simulink model "sgMdl_IO723_CANLoopback"  (R2024b)
settings: Solver=FixedStepAuto  StartTime=0.0  StopTime=inf  RelTol=1e-3
undefined symbols (not defined in the file): sgrestbus
libraries: speedgoatlib_IO723 x3
Description:
  | IO723 - CAN Loopback
settings Model: ModifiedByFormat=Speedgoat  Creator=Speedgoat  LastModifiedBy=Speedgoat
settings SolverCC: ConcurrentTasks=on  PositivePriorityOrder=on
settings OptimizationCC: BlockReduction=off  OptimizeBlockIOStorage=off
settings DebuggingCC: TasksWithSamePriorityMsg=none
settings HardwareCC: ProdBitPerLong=64  ProdLongLongMode=on  ProdHWDeviceType=Intel->x86-64 (Linux 64)
settings RTWCC: Description=Speedgoat Real-Time Target Machine  SystemTargetFile=speedgoat.tlc  TemplateMakefile=slrealtime_default_tmf  Toolchain=Simulink Real-Time Toolchain  BuildConfiguration=Faster Runs  TargetLang=C++
settings SimulinkRealTimeTargetCC: SubcomponentCodeInterfacePackaging=Reusable function  InstructionSetFMA=off  LogToMDFFile=off  SLRTFileLogMaxRuns=10
settings ConfigComp: CovBoundaryAbsTol=1.0e-5

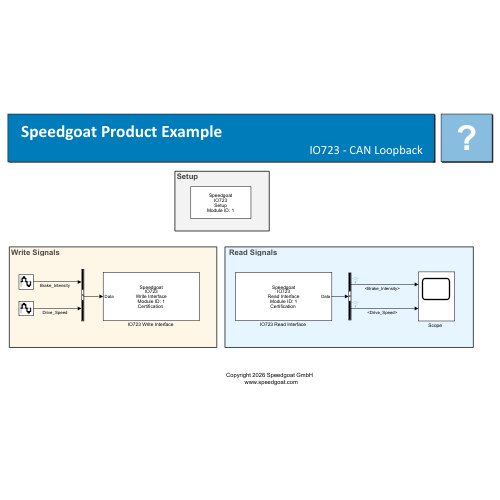
[thumbnail: Simulink's stored preview of the top-level diagram]
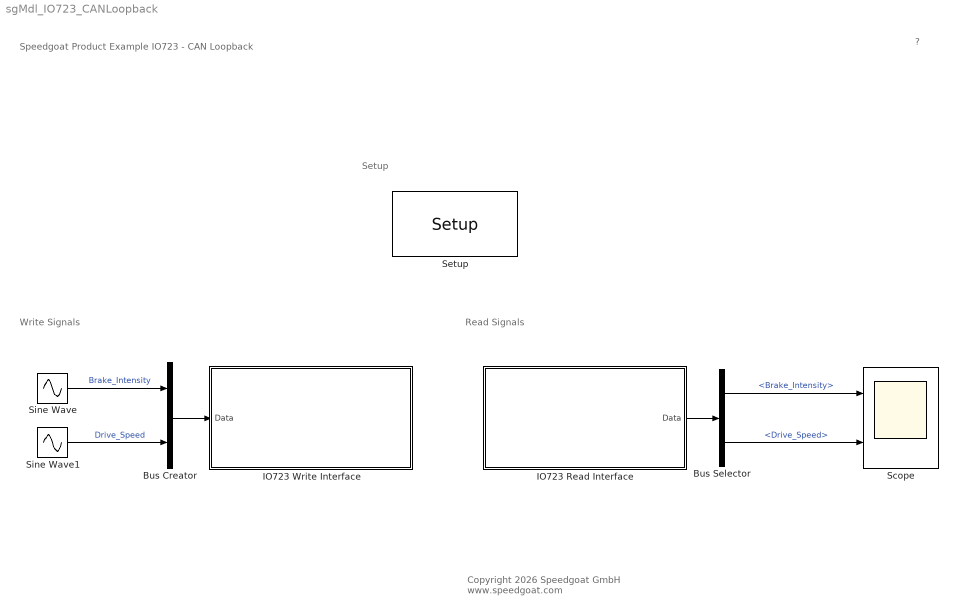
== system sgMdl_IO723_CANLoopback ==
  note: Setup
  note: Write Signals
  note: Read Signals
  note: Speedgoat Product Example
      | IO723 - CAN Loopback
  note: ?
  note: Copyright 2026 Speedgoat GmbH
      |  www.speedgoat.com
  Bus Creator : BusCreator  Inputs=2
  Bus Selector : BusSelector  OutputSignals=CAN1.BRAKE.Brake_frame.Brake_pdu.Brake_Intensity,CAN2.DRIVE.Drive_frame.Drive_pdu.Drive_Speed
  "IO723 Read Interface " : Subsystem  InitFcn=sgrestbus.checkRBSver(gcb);
      settings: OpenFcn=sgrestbus.gui.OpenFcnIO723Interface();
      settings: CopyFcn=|
      | if strcmp(get_param(gcb, 'LinkStatus'), 'resolved')
      |     set_param(gcb, 'LinkStatus', 'breakWithoutHierarchy');
      | end
      mask Help: eval('sg.utils.help.show(''io_main/refentry_io723_read_interface'');')
      mask Display: disp('Speedgoat\nIO723\nRead Interface\nModule ID: 1\nCertification ');
  "IO723 Write Interface " : Subsystem  InitFcn=sgrestbus.checkRBSver(gcb);
      settings: OpenFcn=sgrestbus.gui.OpenFcnIO723Interface();
      settings: CopyFcn=|
      | if strcmp(get_param(gcb, 'LinkStatus'), 'resolved')
      |     set_param(gcb, 'LinkStatus', 'breakWithoutHierarchy');
      | end
      mask Help: eval('sg.utils.help.show(''io_main/refentry_io723_write_interface'');')
      mask Display: disp('Speedgoat\nIO723\nWrite Interface\nModule ID: 1\nCertification ');
  "Scope  " : Scope  NumInputPorts=2
  "Setup " : speedgoatlib_IO723/Setup   parModuleId=1  parPciSlot=-1  parProject='FL3X_CANLoopback\CANLoopback.fcr'  parFPGAver=[16777217 224]  parRBSver='638636542544043106'
  Sine Wave : Sin  Amplitude=10  Bias=10  Frequency=2*pi  SampleTime=0.005
  Sine Wave1 : Sin  Amplitude=20  Bias=20  Frequency=2*pi  SampleTime=0.005
  wires:
  "IO723 Read Interface "/1(Data) -> Bus Selector/1
  Bus Selector/1 -> "Scope  "/1  "<Brake_Intensity>"
  Bus Selector/2 -> "Scope  "/2  "<Drive_Speed>"
  Sine Wave/1 -> Bus Creator/1  "Brake_Intensity"
  Sine Wave1/1 -> Bus Creator/2  "Drive_Speed"
  Bus Creator/1 -> "IO723 Write Interface "/1(Data)

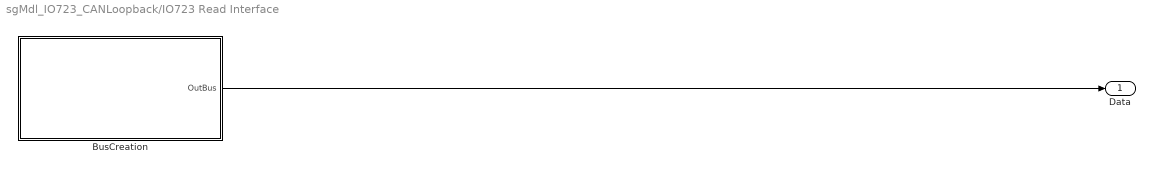
== system sgMdl_IO723_CANLoopback/IO723 Read Interface  ==
  BusCreation : Subsystem
  Data : Outport
  wires:
  BusCreation/1(OutBus) -> Data/1

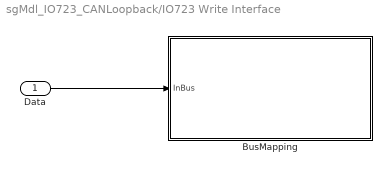
== system sgMdl_IO723_CANLoopback/IO723 Write Interface  ==
  Data : Inport
  BusMapping : Subsystem
  wires:
  Data/1 -> BusMapping/1(InBus)

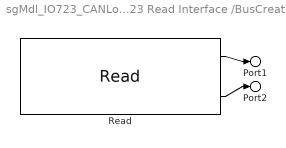
== system sgMdl_IO723_CANLoopback/IO723 Read Interface /BusCreation ==
  "Read " : speedgoatlib_IO723/IO723 Read Interface /Read   parModuleId=1  parSignalId="[2567628  2569300]"  parSignalLen="[8  8]"  parOutType="[0  0]"  parSampleTime=0.005  parPciSlot=-1
  Port1 : Outport  PortName=OutBus  Element=CAN1.BRAKE.Brake_frame.Brake_pdu.Brake_Intensity
  Port2 : Outport  PortName=OutBus  Element=CAN2.DRIVE.Drive_frame.Drive_pdu.Drive_Speed
  wires:
  "Read "/1 -> Port1/1
  "Read "/2 -> Port2/1

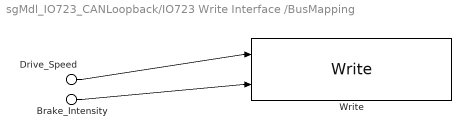
== system sgMdl_IO723_CANLoopback/IO723 Write Interface /BusMapping ==
  Drive_Speed : Inport  PortName=InBus  Element=Drive_Speed
  Brake_Intensity : Inport  PortName=InBus  Element=Brake_Intensity
  "Write " : speedgoatlib_IO723/IO723 Write Interface /Write   parModuleId=1  parSignalId="[2567112  2568784]"  parSignalLen="[8  8]"  parInpType="[0  0]"  parSampleTime=0.005  parPciSlot=-1
  wires:
  Drive_Speed/1 -> "Write "/1
  Brake_Intensity/1 -> "Write "/2
